simulink library "Pitch_Actuation_Linkage_Lib_org"  (Simulink 10.0)
settings: Solver=ode45  StartTime=0.0  StopTime=10.0  RelTol=1e-3  EnableMultiTasking=on
undefined symbols (not defined in the file): WT_Params
libraries: mblibv1 x1
Description:
  | Copyright 2009-2017 The MathWorks, Inc. MathWorks, Inc.
settings Model: Creator=smiller  LastModifiedBy=annonymous

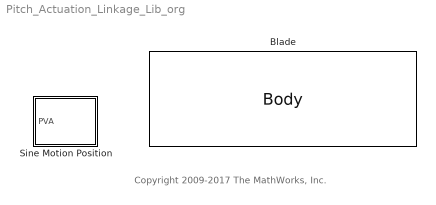
== system Pitch_Actuation_Linkage_Lib_org ==
  note: Copyright 2009-2017 The MathWorks, Inc.
  Blade : mblibv1/Bodies/Body  LConnTagsString=CS4|CS6|CS1|CS5  RConnTagsString=CS2  UpdateFromCAD=off  DialogClass=MechanicalBodyBlock  Mass=WT_Params.Blade.mass  MassUnits=kg  InertiaUnits=kg*m^2  Inertia=WT_Params.Blade.inertia  Shape=Cylinder  ShapeDims=[1 1]  ShapeUnits=m  ShapeUse=false  Density=1  DensityUnits=kg/m^3  DensityUse=false  GraphicsMode=MACHINE_DEFAULT  BodyColorSelMode=COLORPALETTE  BodyColor=[1 1 1]  AttachedToCS=CG  CG=Left$CG$[0 WT_Params.Blade.length/2 0]$CS1$CS1$m$[0 0 0]$Euler X-Y-Z$deg$CS1$false$none  WorkingFrames=Left$CS4$[0 0 0]$CS1$CS1$m$[0 0 0]$Euler X-Y-Z$deg$CS1$true$none#Left$CS6$[WT_Params.Blade.Actuator_Offset.x WT_Params.Blade.Actuator_Offset.y WT_Params.Blade.Actuator_Offset.z]$CS1$CS1$m$[0 0 0]$Euler X-Y-Z$deg$CS1$true$none#Left$CS1$[0 0 0]$Adjoining$Adjoining$m$[0 0 0]$Euler X-Y-Z$deg$Adjoining$true$none#Left$CS7$[WT_Params.Blade.Geometry.root_radius*sin(0) 0 WT_Params.Blade.Geometry.root_radius*cos(0)]$CS1$CS1$m$[0 0 0]$Euler X-Y-Z$deg$CS1$false$none#Left$CS8$[WT_Params.Blade.Geometry.root_radius*sin(0.2*pi) 0 WT_Params.Blade.Geometry.root_radius*cos(0.2*pi)]$CS1$CS1$m$[0 0 0]$Euler X-Y-Z$deg$CS1$false$none#Left$CS9$[WT_Params.Blade.Geometry.root_radius*sin(0.4*pi) 0 WT_Params.Blade.Geometry.root_radius*cos(0.4*pi)]$CS1$CS1$m$[0 0 0]$Euler X-Y-Z$deg$CS1$false$none#Left$CS10$[WT_Params.Blade.Geometry.root_radius*sin(0.6*pi) 0 WT_Params.Blade.Geometry.root_radius*cos(0.6*pi)]$CS1$CS1$m$[0 0 0]$Euler X-Y-Z$deg$CS1$false$none#Left$CS11$[WT_Params.Blade.Geometry.root_radius*sin(0.8*pi) 0 WT_Params.Blade.Geometry.root_radius*cos(0.8*pi)]$CS1$CS1$m$[0 0 0]$Euler X-Y-Z$deg$CS1$false$none#Left$CS12$[WT_Params.Blade.Geometry.root_radius*sin(1.0*pi) 0 WT_Params.Blade.Geometry.root_radius*cos(1.0*pi)]$CS1$CS1$m$[0 0 0]$Euler X-Y-Z$deg$CS1$false$none#Left$CS13$[WT_Params.Blade.Geometry.root_radius*sin(1.2*pi) 0 WT_Params.Blade.Geometry.root_radius*cos(1.2*pi)]$CS1$CS1$m$[0 0 0]$Euler X-Y-Z$deg$CS1$false$none#Left$CS14$[WT_Params.Blade.Geometry.root_radius*sin(1.4*pi) 0 WT_Params.Blade.Geometry.root_radius*cos(1.4*pi)]$CS1$CS1$m$[0 0 0]$Euler X-Y-Z$deg$CS1$false$none#Left$CS15$[WT_Params.Blade.Geometry.root_radius*sin(1.6*pi) 0 WT_Params.Blade.Geometry.root_radius*cos(1.6*pi)]$CS1$CS1$m$[0 0 0]$Euler X-Y-Z$deg$CS1$false$none#Left$CS16$[WT_Params.Blade.Geometry.root_radius*sin(1.8*pi) 0 WT_Params.Blade.Geometry.root_radius*cos(1.8*pi)]$CS1$CS1$m$[0 0 0]$Euler X-Y-Z$deg$CS1$false$none#Left$CS17$[0 WT_Params.Blade.length/4 0]$CS1$CS1$m$[0 0 0]$Euler X-Y-Z$deg$CS1$false$none#Left$CS18$[WT_Params.Blade.Geometry.ctr_to_leading_edge.x 0 WT_Params.Blade.Geometry.ctr_to_leading_edge.z]$CS17$CS17$m$[0 0 0]$Euler X-Y-Z$deg$CS1$false$none#Left$CS19$[WT_Params.Blade.Geometry.ctr_to_a1.x 0 WT_Params.Blade.Geometry.ctr_to_a1.z]$CS17$CS17$m$[0 0 0]$Euler X-Y-Z$deg$CS1$false$none#Left$CS20$[WT_Params.Blade.Geometry.ctr_to_a2.x 0 WT_Params.Blade.Geometry.ctr_to_a2.z]$CS17$CS17$m$[0 0 0]$Euler X-Y-Z$deg$CS1$false$none#Left$CS21$[WT_Params.Blade.Geometry.ctr_to_b1.x 0 WT_Params.Blade.Geometry.ctr_to_b1.z]$CS17$CS17$m$[0 0 0]$Euler X-Y-Z$deg$CS1$false$none#Left$CS25$[WT_Params.Blade.Geometry.ctr_to_b2.x 0 WT_Params.Blade.Geometry.ctr_to_b2.z]$CS17$CS17$m$[0 0 0]$Euler X-Y-Z$deg$CS1$false$none#Left$CS22$[WT_Params.Blade.Geometry.ctr_to_c1.x 0 WT_Params.Blade.Geometry.ctr_to_c1.z]$CS17$CS17$m$[0 0 0]$Euler X-Y-Z$deg$CS1$false$none#Left$CS3$[WT_Params.Blade.Geometry.ctr_to_d1.x 0 WT_Params.Blade.Geometry.ctr_to_d1.z]$CS17$CS17$m$[0 0 0]$Euler X-Y-Z$deg$CS1$false$none#Left$CS23$[WT_Params.Blade.Geometry.ctr_to_e1.x 0 WT_Params.Blade.Geometry.ctr_to_e1.z]$CS17$CS17$m$[0 0 0]$Euler X-Y-Z$deg$CS1$false$none#Left$CS24$[WT_Params.Blade.Geometry.ctr_to_trailing_edge.x 0 WT_Params.Blade.Geometry.ctr_to_trailing_edge.z]$CS17$CS17$m$[0 0 0]$Euler X-Y-Z$deg$CS1$false$none#Left$CS5$[0 0 0]$CS1$CS1$m$[0 0 0]$Euler X-Y-Z$deg$CS1$true$none#Right$CS2$[0 WT_Params.Blade.length 0]$CS1$CS1$m$[0 0 0]$Euler X-Y-Z$deg$CS1$true$none  CGPos=[0 WT_Params.Blade.length/2 0]  CGRot=[0 0 0]  CS0Pos=[]  CS0Rot=[]  CS1Pos=[0 0 0]  CS1Rot=[0 0 0]  CS2Pos=[0 WT_Params.Blade.length 0]  CS2Rot=[0 0 0]  CS3Pos=[WT_Params.Blade.Geometry.ctr_to_d1.x 0 WT_Params.Blade.Geometry.ctr_to_d1.z]  CS3Rot=[0 0 0]  CS4Pos=[0 0 0]  CS4Rot=[0 0 0]  CS5Pos=[0 0 0]  CS5Rot=[0 0 0]  CS6Pos=[WT_Params.Blade.Actuator_Offset.x WT_Params.Blade.Actuator_Offset.y WT_Params.Blade.Actuator_Offset.z]  CS6Rot=[0 0 0]  CS7Pos=[WT_Params.Blade.Geometry.root_radius*sin(0) 0 WT_Params.Blade.Geometry.root_radius*cos(0)]  CS7Rot=[0 0 0]  CS8Pos=[WT_Params.Blade.Geometry.root_radius*sin(0.2*pi) 0 WT_Params.Blade.Geometry.root_radius*cos(0.2*pi)]  CS8Rot=[0 0 0]  CS9Pos=[WT_Params.Blade.Geometry.root_radius*sin(0.4*pi) 0 WT_Params.Blade.Geometry.root_radius*cos(0.4*pi)]  CS9Rot=[0 0 0]  CS10Pos=[WT_Params.Blade.Geometry.root_radius*sin(0.6*pi) 0 WT_Params.Blade.Geometry.root_radius*cos(0.6*pi)]  CS10Rot=[0 0 0]  CS11Pos=[WT_Params.Blade.Geometry.root_radius*sin(0.8*pi) 0 WT_Params.Blade.Geometry.root_radius*cos(0.8*pi)]  CS11Rot=[0 0 0]  CS12Pos=[WT_Params.Blade.Geometry.root_radius*sin(1.0*pi) 0 WT_Params.Blade.Geometry.root_radius*cos(1.0*pi)]  CS12Rot=[0 0 0]  CS13Pos=[WT_Params.Blade.Geometry.root_radius*sin(1.2*pi) 0 WT_Params.Blade.Geometry.root_radius*cos(1.2*pi)]  CS13Rot=[0 0 0]  CS14Pos=[WT_Params.Blade.Geometry.root_radius*sin(1.4*pi) 0 WT_Params.Blade.Geometry.root_radius*cos(1.4*pi)]  CS14Rot=[0 0 0]  CS15Pos=[WT_Params.Blade.Geometry.root_radius*sin(1.6*pi) 0 WT_Params.Blade.Geometry.root_radius*cos(1.6*pi)]  CS15Rot=[0 0 0]  CS16Pos=[WT_Params.Blade.Geometry.root_radius*sin(1.8*pi) 0 WT_Params.Blade.Geometry.root_radius*cos(1.8*pi)]  CS16Rot=[0 0 0]  CS17Pos=[0 WT_Params.Blade.length/4 0]  CS17Rot=[0 0 0]  CS18Pos=[WT_Params.Blade.Geometry.ctr_to_leading_edge.x 0 WT_Params.Blade.Geometry.ctr_to_leading_edge.z]  CS18Rot=[0 0 0]  CS19Pos=[WT_Params.Blade.Geometry.ctr_to_a1.x 0 WT_Params.Blade.Geometry.ctr_to_a1.z]  CS19Rot=[0 0 0]  CS20Pos=[WT_Params.Blade.Geometry.ctr_to_a2.x 0 WT_Params.Blade.Geometry.ctr_to_a2.z]  CS20Rot=[0 0 0]
      settings: SourceProductName=Simscape Multibody  SourceProductBaseCode=MS
  Sine Motion Position : Subsystem  mask{Amplitude=0.2, pd=5, PhaseShift=0}
      mask prompts: pd "Period (Seconds)"; PhaseShift "Phase Shift (Degrees)"

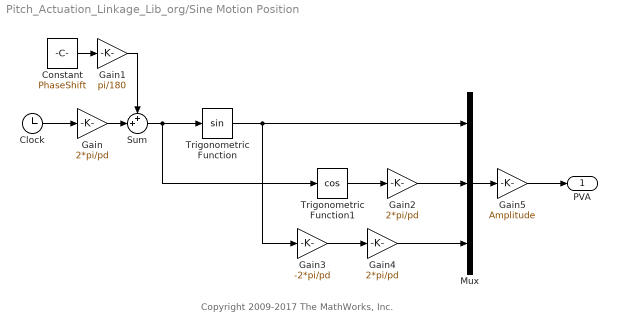
== system Pitch_Actuation_Linkage_Lib_org/Sine Motion Position ==
  note: Copyright 2009-2017 The MathWorks, Inc.
  Clock : Clock
  Constant : Constant  Value=PhaseShift
  Gain : Gain  Gain=2*pi/pd
  Gain1 : Gain  Gain=pi/180
  Gain2 : Gain  Gain=2*pi/pd
  Gain3 : Gain  Gain=-2*pi/pd
  Gain4 : Gain  Gain=2*pi/pd
  Gain5 : Gain  Gain=Amplitude
  Mux : Mux  Inputs=3
  Sum : Sum  Inputs=++|
  Trigonometric Function : Trigonometry
  Trigonometric Function1 : Trigonometry  Operator=cos
  PVA : Outport
  wires:
  Gain4/1 -> Mux/3
  Gain3/1 -> Gain4/1
  Gain2/1 -> Mux/2
  Trigonometric Function1/1 -> Gain2/1
  Gain5/1 -> PVA/1
  Mux/1 -> Gain5/1
  Trigonometric Function/1 -> Gain3/1, Mux/1
  Sum/1 -> Trigonometric Function1/1, Trigonometric Function/1
  Gain1/1 -> Sum/1
  Constant/1 -> Gain1/1
  Gain/1 -> Sum/2
  Clock/1 -> Gain/1
